simulink library "relay_housing_lib"  (Simulink 8.1)
settings: Solver=ode45  StartTime=0.0  StopTime=10.0  RelTol=1e-3
values from neighbouring files (symbols this model uses):
  Ts = 100E-6    (= 0.0001)    [BANSHEE_init.m]
undefined symbols (not defined in the file or in its folder): F1, F2, F3, generic_ethernet_cb
libraries: relay_modbus_lib x42, rtio_generic_modbus x42, rtlab x5, udp_powerfactor_lib x3, PQFV_lib x3, opal_lib x1, DMS_slave_lib x1, LoadProfiles_lib x1
(part 1 of 2)
settings Model: Creator=re25624  LastModifiedBy=g73labuser

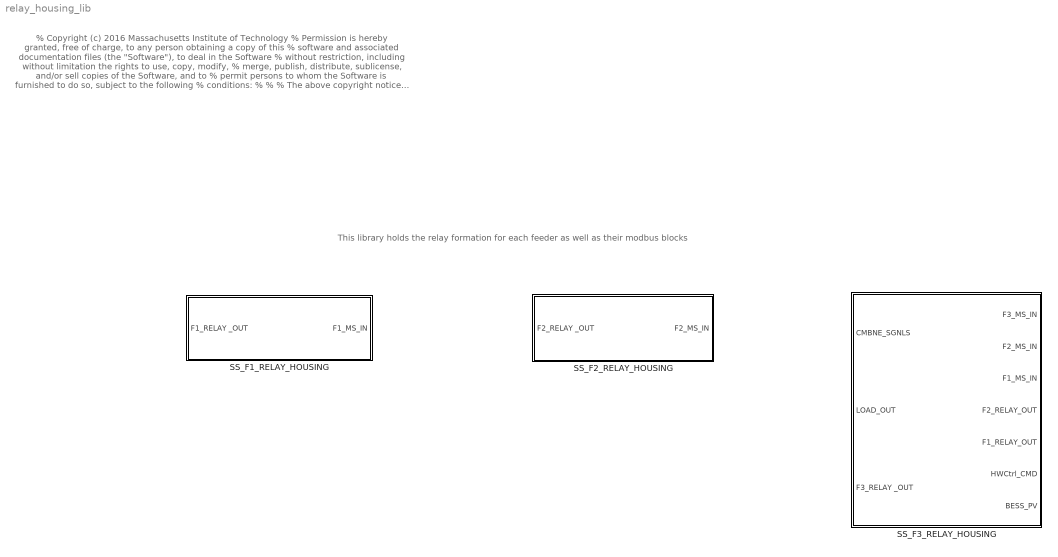
== system relay_housing_lib ==
  note: This library holds the relay formation for each feeder as well as their modbus blocks
  note: % Copyright (c) 2016 Massachusetts Institute of Technology
      | % Permission is hereby granted, free of charge, to any person obtaining a copy of this
      | % software and associated documentation files (the "Software"), to deal in the Software
      | % without restriction, including without limitation the rights to use, copy, modify,
      | % merge, publish, distribute, sublicense, and/or sell copies of the Software, and to
      | % permit persons to whom the Software is furnished to do so, subject to the following
      | % conditions:
      | %
      | %
      | % The above copyright notice and this permission notice shall be included in
      | % all copies or substantial portions of the Software.
      | %
      | % THE SOFTWARE IS PROVIDED "AS IS", WITHOUT WARRANTY OF ANY KIND, EXPRESS OR IMPLIED,
      | % INCLUDING BUT NOT LIMITED TO THE WARRANTIES OF MERCHANTABILITY, FITNESS FOR A
      | % PARTICULAR PURPOSE AND NONINFRINGEMENT. IN NO EVENT SHALL THE AUTHORS OR COPYRIGHT
      | % HOLDERS BE LIABLE FOR ANY CLAIM, DAMAGES OR OTHER LIABILITY, WHETHER IN AN ACTION
      | % OF CONTRACT, TORT OR OTHERWISE, ARISING FROM, OUT OF OR IN CONNECTION WITH THE
      | % SOFTWARE OR THE USE OR OTHER DEALINGS IN THE SOFTWARE.
      | %
      | %
      | %%
  SS_F1_RELAY_HOUSING : Subsystem
  SS_F2_RELAY_HOUSING : Subsystem
  SS_F3_RELAY_HOUSING : Subsystem

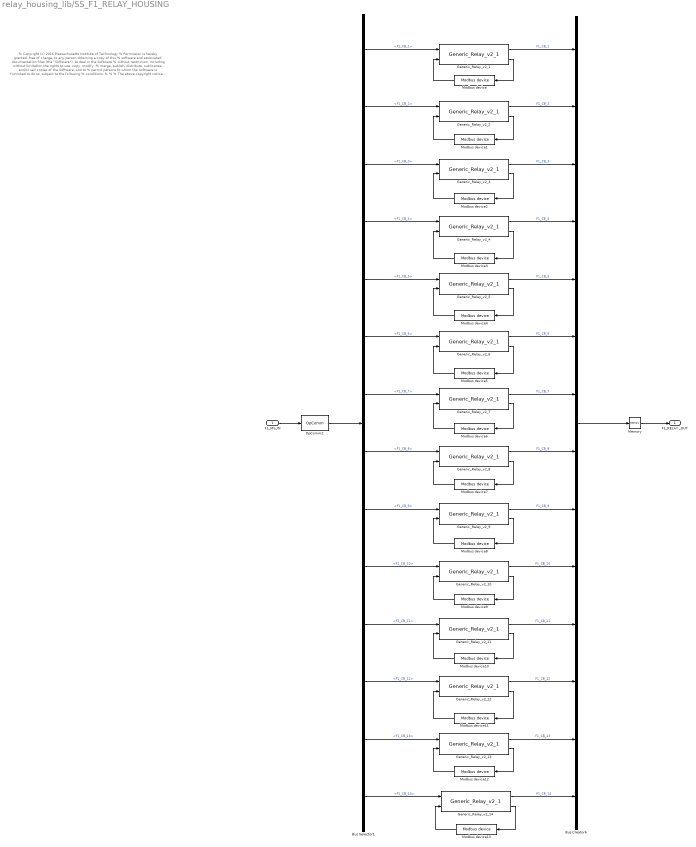
== system relay_housing_lib/SS_F1_RELAY_HOUSING ==
  note: % Copyright (c) 2016 Massachusetts Institute of Technology
      | % Permission is hereby granted, free of charge, to any person obtaining a copy of this
      | % software and associated documentation files (the "Software"), to deal in the Software
      | % without restriction, including without limitation the rights to use, copy, modify,
      | % merge, publish, distribute, sublicense, and/or sell copies of the Software, and to
      | % permit persons to whom the Software is furnished to do so, subject to the following
      | % conditions:
      | %
      | %
      | % The above copyright notice and this permission notice shall be included in
      | % all copies or substantial portions of the Software.
      | %
      | % THE SOFTWARE IS PROVIDED "AS IS", WITHOUT WARRANTY OF ANY KIND, EXPRESS OR IMPLIED,
      | % INCLUDING BUT NOT LIMITED TO THE WARRANTIES OF MERCHANTABILITY, FITNESS FOR A
      | % PARTICULAR PURPOSE AND NONINFRINGEMENT. IN NO EVENT SHALL THE AUTHORS OR COPYRIGHT
      | % HOLDERS BE LIABLE FOR ANY CLAIM, DAMAGES OR OTHER LIABILITY, WHETHER IN AN ACTION
      | % OF CONTRACT, TORT OR OTHERWISE, ARISING FROM, OUT OF OR IN CONNECTION WITH THE
      | % SOFTWARE OR THE USE OR OTHER DEALINGS IN THE SOFTWARE.
      | %
      | %
      | %%
  F1_MS_IN : Inport
  Bus Creator6 : BusCreator  Inputs=14
  Bus Selector1 : BusSelector  OutputSignals=CB_DATA.F1_CB_1,CB_DATA.F1_CB_2,CB_DATA.F1_CB_3,CB_DATA.F1_CB_4,CB_DATA.F1_CB_5,CB_DATA.F1_CB_6,CB_DATA.F1_CB_7,CB_DATA.F1_CB_8,CB_DATA.F1_CB_9,CB_DATA.F1_CB_10,CB_DATA.F1_CB_11,CB_DATA.F1_CB_12,CB_DATA.F1_CB_13,CB_DATA.F1_CB_14
  Generic_Relay_v2_1 : relay_modbus_lib/Generic_Relay_v2_1  Ts=Ts  relay_settings=[F1(1,:)]
  Generic_Relay_v2_10 : relay_modbus_lib/Generic_Relay_v2_1  Ts=Ts  relay_settings=[F1(10,:)]
  Generic_Relay_v2_11 : relay_modbus_lib/Generic_Relay_v2_1  Ts=Ts  relay_settings=[F1(11,:)]
  Generic_Relay_v2_12 : relay_modbus_lib/Generic_Relay_v2_1  Ts=Ts  relay_settings=[F1(12,:)]
  Generic_Relay_v2_13 : relay_modbus_lib/Generic_Relay_v2_1  Ts=Ts  relay_settings=[F1(13,:)]
  Generic_Relay_v2_14 : relay_modbus_lib/Generic_Relay_v2_1  Ts=Ts  relay_settings=[F1(14,:)]
  Generic_Relay_v2_2 : relay_modbus_lib/Generic_Relay_v2_1  Ts=Ts  relay_settings=[F1(2,:)]
  Generic_Relay_v2_3 : relay_modbus_lib/Generic_Relay_v2_1  Ts=Ts  relay_settings=[F1(3,:)]
  Generic_Relay_v2_4 : relay_modbus_lib/Generic_Relay_v2_1  Ts=Ts  relay_settings=[F1(4,:)]
  Generic_Relay_v2_5 : relay_modbus_lib/Generic_Relay_v2_1  Ts=Ts  relay_settings=[F1(5,:)]
  Generic_Relay_v2_6 : relay_modbus_lib/Generic_Relay_v2_1  Ts=Ts  relay_settings=[F1(6,:)]
  Generic_Relay_v2_7 : relay_modbus_lib/Generic_Relay_v2_1  Ts=Ts  relay_settings=[F1(7,:)]
  Generic_Relay_v2_8 : relay_modbus_lib/Generic_Relay_v2_1  Ts=Ts  relay_settings=[F1(8,:)]
  Generic_Relay_v2_9 : relay_modbus_lib/Generic_Relay_v2_1  Ts=Ts  relay_settings=[F1(9,:)]
  Memory : Memory
  Modbus device : rtio_generic_modbus/Modbus device  conf_name=F1_relay_cfg1.opal  conf_name_mask=F1_relay_cfg1.xls  sample_time=Ts
  Modbus device1 : rtio_generic_modbus/Modbus device  conf_name=F1_relay_cfg2.opal  conf_name_mask=F1_relay_cfg2.xls  sample_time=Ts
  Modbus device10 : rtio_generic_modbus/Modbus device  conf_name=F1_relay_cfg11.opal  conf_name_mask=F1_relay_cfg11.xls  sample_time=Ts
  Modbus device11 : rtio_generic_modbus/Modbus device  conf_name=F1_relay_cfg12.opal  conf_name_mask=F1_relay_cfg12.xls  sample_time=Ts
  Modbus device12 : rtio_generic_modbus/Modbus device  conf_name=F1_relay_cfg13.opal  conf_name_mask=F1_relay_cfg13.xls  sample_time=Ts
  Modbus device13 : rtio_generic_modbus/Modbus device  conf_name=F1_relay_cfg14.opal  conf_name_mask=F1_relay_cfg14.xls  sample_time=Ts
  Modbus device2 : rtio_generic_modbus/Modbus device  conf_name=F1_relay_cfg3.opal  conf_name_mask=F1_relay_cfg3.xls  sample_time=Ts
  Modbus device3 : rtio_generic_modbus/Modbus device  conf_name=F1_relay_cfg4.opal  conf_name_mask=F1_relay_cfg4.xls  sample_time=Ts
  Modbus device4 : rtio_generic_modbus/Modbus device  conf_name=F1_relay_cfg5.opal  conf_name_mask=F1_relay_cfg5.xls  sample_time=Ts
  Modbus device5 : rtio_generic_modbus/Modbus device  conf_name=F1_relay_cfg6.opal  conf_name_mask=F1_relay_cfg6.xls  sample_time=Ts
  Modbus device6 : rtio_generic_modbus/Modbus device  conf_name=F1_relay_cfg7.opal  conf_name_mask=F1_relay_cfg7.xls  sample_time=Ts
  Modbus device7 : rtio_generic_modbus/Modbus device  conf_name=F1_relay_cfg8.opal  conf_name_mask=F1_relay_cfg8.xls  sample_time=Ts
  Modbus device8 : rtio_generic_modbus/Modbus device  conf_name=F1_relay_cfg9.opal  conf_name_mask=F1_relay_cfg9.xls  sample_time=Ts
  Modbus device9 : rtio_generic_modbus/Modbus device  conf_name=F1_relay_cfg10.opal  conf_name_mask=F1_relay_cfg10.xls  sample_time=Ts
  OpComm2 : rtlab/OpComm  nbport=1  groupe_acq=1  subsys_rate=0  st=0  Synchronization=on  Interpolation=on  Threshold=1.0  Missed_Data=off  Sim_Time=off  Samples=off  dynSigOut=off  from_console=0  warning_done=off  writeOpCommFile=off  Offset=off
  F1_RELAY _OUT : Outport
  wires:
  Memory/1 -> F1_RELAY _OUT/1
  Bus Selector1/14 -> Generic_Relay_v2_14/1  "<F1_CB_14>"
  Generic_Relay_v2_14/1 -> Bus Creator6/14  "F1_CB_14"
  Generic_Relay_v2_14/2 -> Modbus device13/1
  Modbus device13/1 -> Generic_Relay_v2_14/2
  Generic_Relay_v2_3/1 -> Bus Creator6/3  "F1_CB_3"
  Generic_Relay_v2_4/1 -> Bus Creator6/4  "F1_CB_4"
  Generic_Relay_v2_5/1 -> Bus Creator6/5  "F1_CB_5"
  Generic_Relay_v2_6/1 -> Bus Creator6/6  "F1_CB_6"
  Generic_Relay_v2_7/1 -> Bus Creator6/7  "F1_CB_7"
  Generic_Relay_v2_8/1 -> Bus Creator6/8  "F1_CB_8"
  Generic_Relay_v2_9/1 -> Bus Creator6/9  "F1_CB_9"
  Generic_Relay_v2_10/1 -> Bus Creator6/10  "F1_CB_10"
  Generic_Relay_v2_11/1 -> Bus Creator6/11  "F1_CB_11"
  Generic_Relay_v2_12/1 -> Bus Creator6/12  "F1_CB_12"
  Generic_Relay_v2_13/1 -> Bus Creator6/13  "F1_CB_13"
  Bus Selector1/13 -> Generic_Relay_v2_13/1  "<F1_CB_13>"
  Bus Selector1/12 -> Generic_Relay_v2_12/1  "<F1_CB_12>"
  Bus Selector1/11 -> Generic_Relay_v2_11/1  "<F1_CB_11>"
  Bus Selector1/10 -> Generic_Relay_v2_10/1  "<F1_CB_10>"
  Bus Selector1/9 -> Generic_Relay_v2_9/1  "<F1_CB_9>"
  Bus Selector1/8 -> Generic_Relay_v2_8/1  "<F1_CB_8>"
  Bus Selector1/7 -> Generic_Relay_v2_7/1  "<F1_CB_7>"
  Bus Selector1/6 -> Generic_Relay_v2_6/1  "<F1_CB_6>"
  Bus Selector1/5 -> Generic_Relay_v2_5/1  "<F1_CB_5>"
  Bus Selector1/4 -> Generic_Relay_v2_4/1  "<F1_CB_4>"
  Bus Selector1/3 -> Generic_Relay_v2_3/1  "<F1_CB_3>"
  Generic_Relay_v2_2/1 -> Bus Creator6/2  "F1_CB_2"
  Bus Selector1/2 -> Generic_Relay_v2_2/1  "<F1_CB_2>"
  Bus Creator6/1 -> Memory/1
  Generic_Relay_v2_1/1 -> Bus Creator6/1  "F1_CB_1"
  Bus Selector1/1 -> Generic_Relay_v2_1/1  "<F1_CB_1>"
  F1_MS_IN/1 -> OpComm2/1
  Modbus device/1 -> Generic_Relay_v2_1/2
  Generic_Relay_v2_1/2 -> Modbus device/1
  Modbus device1/1 -> Generic_Relay_v2_2/2
  Generic_Relay_v2_2/2 -> Modbus device1/1
  Generic_Relay_v2_3/2 -> Modbus device2/1
  Modbus device2/1 -> Generic_Relay_v2_3/2
  Generic_Relay_v2_4/2 -> Modbus device3/1
  Modbus device3/1 -> Generic_Relay_v2_4/2
  Generic_Relay_v2_5/2 -> Modbus device4/1
  Modbus device4/1 -> Generic_Relay_v2_5/2
  Generic_Relay_v2_6/2 -> Modbus device5/1
  Modbus device5/1 -> Generic_Relay_v2_6/2
  Generic_Relay_v2_7/2 -> Modbus device6/1
  Modbus device6/1 -> Generic_Relay_v2_7/2
  Generic_Relay_v2_8/2 -> Modbus device7/1
  Modbus device7/1 -> Generic_Relay_v2_8/2
  Generic_Relay_v2_9/2 -> Modbus device8/1
  Modbus device8/1 -> Generic_Relay_v2_9/2
  Generic_Relay_v2_10/2 -> Modbus device9/1
  Modbus device9/1 -> Generic_Relay_v2_10/2
  Generic_Relay_v2_11/2 -> Modbus device10/1
  Modbus device10/1 -> Generic_Relay_v2_11/2
  Generic_Relay_v2_12/2 -> Modbus device11/1
  Modbus device11/1 -> Generic_Relay_v2_12/2
  Generic_Relay_v2_13/2 -> Modbus device12/1
  Modbus device12/1 -> Generic_Relay_v2_13/2
  OpComm2/1 -> Bus Selector1/1

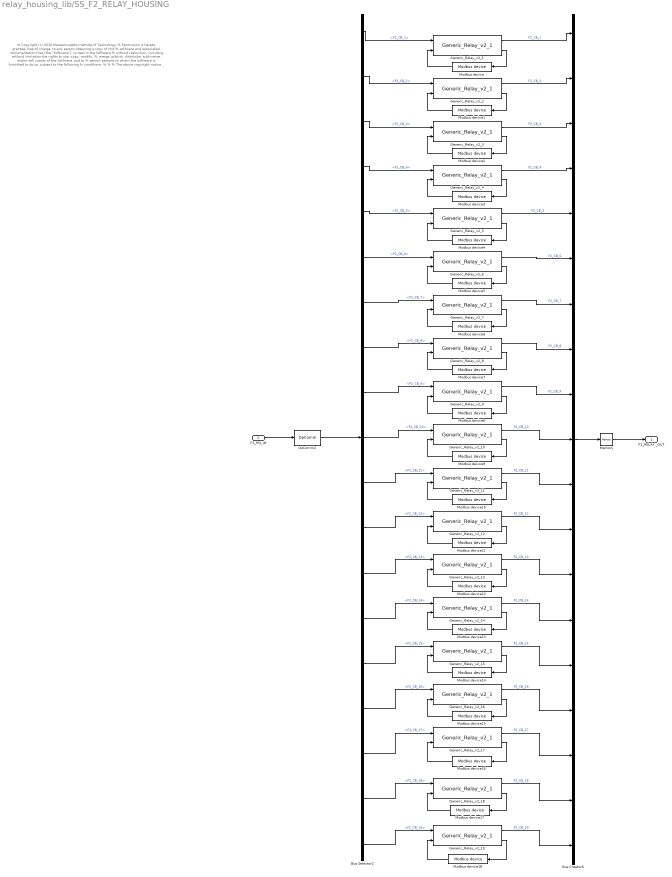
== system relay_housing_lib/SS_F2_RELAY_HOUSING ==
  note: % Copyright (c) 2016 Massachusetts Institute of Technology
      | % Permission is hereby granted, free of charge, to any person obtaining a copy of this
      | % software and associated documentation files (the "Software"), to deal in the Software
      | % without restriction, including without limitation the rights to use, copy, modify,
      | % merge, publish, distribute, sublicense, and/or sell copies of the Software, and to
      | % permit persons to whom the Software is furnished to do so, subject to the following
      | % conditions:
      | %
      | %
      | % The above copyright notice and this permission notice shall be included in
      | % all copies or substantial portions of the Software.
      | %
      | % THE SOFTWARE IS PROVIDED "AS IS", WITHOUT WARRANTY OF ANY KIND, EXPRESS OR IMPLIED,
      | % INCLUDING BUT NOT LIMITED TO THE WARRANTIES OF MERCHANTABILITY, FITNESS FOR A
      | % PARTICULAR PURPOSE AND NONINFRINGEMENT. IN NO EVENT SHALL THE AUTHORS OR COPYRIGHT
      | % HOLDERS BE LIABLE FOR ANY CLAIM, DAMAGES OR OTHER LIABILITY, WHETHER IN AN ACTION
      | % OF CONTRACT, TORT OR OTHERWISE, ARISING FROM, OUT OF OR IN CONNECTION WITH THE
      | % SOFTWARE OR THE USE OR OTHER DEALINGS IN THE SOFTWARE.
      | %
      | %
      | %%
  F2_MS_IN : Inport
  Bus Creator6 : BusCreator  Inputs=19
  Bus Selector2 : BusSelector  OutputSignals=CB_DATA.F2_CB_1,CB_DATA.F2_CB_2,CB_DATA.F2_CB_3,CB_DATA.F2_CB_4,CB_DATA.F2_CB_5,CB_DATA.F2_CB_6,CB_DATA.F2_CB_7,CB_DATA.F2_CB_8,CB_DATA.F2_CB_9,CB_DATA.F2_CB_10,CB_DATA.F2_CB_11,CB_DATA.F2_CB_12,CB_DATA.F2_CB_13,CB_DATA.F2_CB_14,CB_DATA.F2_CB_15,CB_DATA.F2_CB_16,CB_DATA.F2_CB_17,CB_DATA.F2_CB_18,CB_DATA.F2_CB_19
  Generic_Relay_v2_1 : relay_modbus_lib/Generic_Relay_v2_1  Ts=Ts  relay_settings=[F2(1,:)]
  Generic_Relay_v2_10 : relay_modbus_lib/Generic_Relay_v2_1  Ts=Ts  relay_settings=[F2(10,:)]
  Generic_Relay_v2_11 : relay_modbus_lib/Generic_Relay_v2_1  Ts=Ts  relay_settings=[F2(11,:)]
  Generic_Relay_v2_12 : relay_modbus_lib/Generic_Relay_v2_1  Ts=Ts  relay_settings=[F2(12,:)]
  Generic_Relay_v2_13 : relay_modbus_lib/Generic_Relay_v2_1  Ts=Ts  relay_settings=[F2(13,:)]
  Generic_Relay_v2_14 : relay_modbus_lib/Generic_Relay_v2_1  Ts=Ts  relay_settings=[F2(14,:)]
  Generic_Relay_v2_15 : relay_modbus_lib/Generic_Relay_v2_1  Ts=Ts  relay_settings=[F2(15,:)]
  Generic_Relay_v2_16 : relay_modbus_lib/Generic_Relay_v2_1  Ts=Ts  relay_settings=[F2(16,:)]
  Generic_Relay_v2_17 : relay_modbus_lib/Generic_Relay_v2_1  Ts=Ts  relay_settings=[F2(17,:)]
  Generic_Relay_v2_18 : relay_modbus_lib/Generic_Relay_v2_1  Ts=Ts  relay_settings=[F2(18,:)]
  Generic_Relay_v2_19 : relay_modbus_lib/Generic_Relay_v2_1  Ts=Ts  relay_settings=[F2(19,:)]
  Generic_Relay_v2_2 : relay_modbus_lib/Generic_Relay_v2_1  Ts=Ts  relay_settings=[F2(2,:)]
  Generic_Relay_v2_3 : relay_modbus_lib/Generic_Relay_v2_1  Ts=Ts  relay_settings=[F2(3,:)]
  Generic_Relay_v2_4 : relay_modbus_lib/Generic_Relay_v2_1  Ts=Ts  relay_settings=[F2(4,:)]
  Generic_Relay_v2_5 : relay_modbus_lib/Generic_Relay_v2_1  Ts=Ts  relay_settings=[F2(5,:)]
  Generic_Relay_v2_6 : relay_modbus_lib/Generic_Relay_v2_1  Ts=Ts  relay_settings=[F2(6,:)]
  Generic_Relay_v2_7 : relay_modbus_lib/Generic_Relay_v2_1  Ts=Ts  relay_settings=[F2(7,:)]
  Generic_Relay_v2_8 : relay_modbus_lib/Generic_Relay_v2_1  Ts=Ts  relay_settings=[F2(8,:)]
  Generic_Relay_v2_9 : relay_modbus_lib/Generic_Relay_v2_1  Ts=Ts  relay_settings=[F2(9,:)]
  Memory : Memory
  Modbus device : rtio_generic_modbus/Modbus device  conf_name=F2_relay_cfg1.opal  conf_name_mask=F2_relay_cfg1.xls  sample_time=Ts
  Modbus device1 : rtio_generic_modbus/Modbus device  conf_name=F2_relay_cfg2.opal  conf_name_mask=F2_relay_cfg2.xls  sample_time=Ts
  Modbus device10 : rtio_generic_modbus/Modbus device  conf_name=F2_relay_cfg11.opal  conf_name_mask=F2_relay_cfg11.xls  sample_time=Ts
  Modbus device11 : rtio_generic_modbus/Modbus device  conf_name=F2_relay_cfg12.opal  conf_name_mask=F2_relay_cfg12.xls  sample_time=Ts
  Modbus device12 : rtio_generic_modbus/Modbus device  conf_name=F2_relay_cfg13.opal  conf_name_mask=F2_relay_cfg13.xls  sample_time=Ts
  Modbus device13 : rtio_generic_modbus/Modbus device  conf_name=F2_relay_cfg14.opal  conf_name_mask=F2_relay_cfg14.xls  sample_time=Ts
  Modbus device14 : rtio_generic_modbus/Modbus device  conf_name=F2_relay_cfg15.opal  conf_name_mask=F2_relay_cfg15.xls  sample_time=Ts
  Modbus device15 : rtio_generic_modbus/Modbus device  conf_name=F2_relay_cfg16.opal  conf_name_mask=F2_relay_cfg16.xls  sample_time=Ts
  Modbus device16 : rtio_generic_modbus/Modbus device  conf_name=F2_relay_cfg17.opal  conf_name_mask=F2_relay_cfg17.xls  sample_time=Ts
  Modbus device17 : rtio_generic_modbus/Modbus device  conf_name=F2_relay_cfg18.opal  conf_name_mask=F2_relay_cfg18.xls  sample_time=Ts
  Modbus device18 : rtio_generic_modbus/Modbus device  conf_name=F2_relay_cfg19.opal  conf_name_mask=F2_relay_cfg19.xls  sample_time=Ts
  Modbus device2 : rtio_generic_modbus/Modbus device  conf_name=F2_relay_cfg3.opal  conf_name_mask=F2_relay_cfg3.xls  sample_time=Ts
  Modbus device3 : rtio_generic_modbus/Modbus device  conf_name=F2_relay_cfg4.opal  conf_name_mask=F2_relay_cfg4.xls  sample_time=Ts
  Modbus device4 : rtio_generic_modbus/Modbus device  conf_name=F2_relay_cfg5.opal  conf_name_mask=F2_relay_cfg5.xls  sample_time=Ts
  Modbus device5 : rtio_generic_modbus/Modbus device  conf_name=F2_relay_cfg6.opal  conf_name_mask=F2_relay_cfg6.xls  sample_time=Ts
  Modbus device6 : rtio_generic_modbus/Modbus device  conf_name=F2_relay_cfg7.opal  conf_name_mask=F2_relay_cfg7.xls  sample_time=Ts
  Modbus device7 : rtio_generic_modbus/Modbus device  conf_name=F2_relay_cfg8.opal  conf_name_mask=F2_relay_cfg8.xls  sample_time=Ts
  Modbus device8 : rtio_generic_modbus/Modbus device  conf_name=F2_relay_cfg9.opal  conf_name_mask=F2_relay_cfg9.xls  sample_time=Ts
  Modbus device9 : rtio_generic_modbus/Modbus device  conf_name=F2_relay_cfg10.opal  conf_name_mask=F2_relay_cfg10.xls  sample_time=Ts
  OpComm2 : rtlab/OpComm  nbport=1  groupe_acq=1  subsys_rate=0  st=0  Synchronization=on  Interpolation=on  Threshold=1.0  Missed_Data=off  Sim_Time=off  Samples=off  dynSigOut=off  from_console=0  warning_done=off  writeOpCommFile=off  Offset=off
  F2_RELAY _OUT : Outport
  wires:
  Memory/1 -> F2_RELAY _OUT/1
  Bus Selector2/18 -> Generic_Relay_v2_18/1  "<F2_CB_18>"
  Bus Selector2/19 -> Generic_Relay_v2_19/1  "<F2_CB_19>"
  Generic_Relay_v2_19/1 -> Bus Creator6/19  "F2_CB_19"
  Generic_Relay_v2_18/1 -> Bus Creator6/18  "F2_CB_18"
  Generic_Relay_v2_18/2 -> Modbus device17/1
  Modbus device17/1 -> Generic_Relay_v2_18/2
  Generic_Relay_v2_19/2 -> Modbus device18/1
  Modbus device18/1 -> Generic_Relay_v2_19/2
  Bus Selector2/17 -> Generic_Relay_v2_17/1  "<F2_CB_17>"
  Generic_Relay_v2_17/1 -> Bus Creator6/17  "F2_CB_17"
  Generic_Relay_v2_6/1 -> Bus Creator6/6  "F2_CB_6"
  Generic_Relay_v2_5/1 -> Bus Creator6/5  "F2_CB_5"
  Generic_Relay_v2_4/1 -> Bus Creator6/4  "F2_CB_4"
  Generic_Relay_v2_3/1 -> Bus Creator6/3  "F2_CB_3"
  Generic_Relay_v2_2/1 -> Bus Creator6/2  "F2_CB_2"
  Generic_Relay_v2_7/1 -> Bus Creator6/7  "F2_CB_7"
  Generic_Relay_v2_8/1 -> Bus Creator6/8  "F2_CB_8"
  Generic_Relay_v2_9/1 -> Bus Creator6/9  "F2_CB_9"
  Generic_Relay_v2_10/1 -> Bus Creator6/10  "F2_CB_10"
  Generic_Relay_v2_11/1 -> Bus Creator6/11  "F2_CB_11"
  Generic_Relay_v2_16/1 -> Bus Creator6/16  "F2_CB_16"
  Generic_Relay_v2_15/1 -> Bus Creator6/15  "F2_CB_15"
  Generic_Relay_v2_14/1 -> Bus Creator6/14  "F2_CB_14"
  Generic_Relay_v2_13/1 -> Bus Creator6/13  "F2_CB_13"
  Generic_Relay_v2_12/1 -> Bus Creator6/12  "F2_CB_12"
  Bus Selector2/16 -> Generic_Relay_v2_16/1  "<F2_CB_16>"
  Bus Selector2/15 -> Generic_Relay_v2_15/1  "<F2_CB_15>"
  Bus Selector2/14 -> Generic_Relay_v2_14/1  "<F2_CB_14>"
  Bus Selector2/13 -> Generic_Relay_v2_13/1  "<F2_CB_13>"
  Bus Selector2/12 -> Generic_Relay_v2_12/1  "<F2_CB_12>"
  Bus Selector2/11 -> Generic_Relay_v2_11/1  "<F2_CB_11>"
  Bus Selector2/10 -> Generic_Relay_v2_10/1  "<F2_CB_10>"
  Bus Selector2/9 -> Generic_Relay_v2_9/1  "<F2_CB_9>"
  Bus Selector2/8 -> Generic_Relay_v2_8/1  "<F2_CB_8>"
  Bus Selector2/7 -> Generic_Relay_v2_7/1  "<F2_CB_7>"
  Bus Selector2/6 -> Generic_Relay_v2_6/1  "<F2_CB_6>"
  Bus Selector2/5 -> Generic_Relay_v2_5/1  "<F2_CB_5>"
  Bus Selector2/4 -> Generic_Relay_v2_4/1  "<F2_CB_4>"
  Bus Selector2/3 -> Generic_Relay_v2_3/1  "<F2_CB_3>"
  Bus Selector2/2 -> Generic_Relay_v2_2/1  "<F2_CB_2>"
  Generic_Relay_v2_1/1 -> Bus Creator6/1  "F2_CB_1"
  Bus Selector2/1 -> Generic_Relay_v2_1/1  "<F2_CB_1>"
  F2_MS_IN/1 -> OpComm2/1
  Bus Creator6/1 -> Memory/1
  Generic_Relay_v2_1/2 -> Modbus device/1
  Modbus device/1 -> Generic_Relay_v2_1/2
  Generic_Relay_v2_2/2 -> Modbus device1/1
  Modbus device1/1 -> Generic_Relay_v2_2/2
  Generic_Relay_v2_3/2 -> Modbus device2/1
  Modbus device2/1 -> Generic_Relay_v2_3/2
  Generic_Relay_v2_4/2 -> Modbus device3/1
  Modbus device3/1 -> Generic_Relay_v2_4/2
  Generic_Relay_v2_5/2 -> Modbus device4/1
  Modbus device4/1 -> Generic_Relay_v2_5/2
  Modbus device5/1 -> Generic_Relay_v2_6/2
  Generic_Relay_v2_6/2 -> Modbus device5/1
  Generic_Relay_v2_7/2 -> Modbus device6/1
  Modbus device6/1 -> Generic_Relay_v2_7/2
  Generic_Relay_v2_8/2 -> Modbus device7/1
  Modbus device7/1 -> Generic_Relay_v2_8/2
  Generic_Relay_v2_9/2 -> Modbus device8/1
  Modbus device8/1 -> Generic_Relay_v2_9/2
  Generic_Relay_v2_10/2 -> Modbus device9/1
  Modbus device9/1 -> Generic_Relay_v2_10/2
  Generic_Relay_v2_11/2 -> Modbus device10/1
  Modbus device10/1 -> Generic_Relay_v2_11/2
  Generic_Relay_v2_12/2 -> Modbus device11/1
  Modbus device11/1 -> Generic_Relay_v2_12/2
  Modbus device12/1 -> Generic_Relay_v2_13/2
  Generic_Relay_v2_13/2 -> Modbus device12/1
  Generic_Relay_v2_14/2 -> Modbus device13/1
  Modbus device13/1 -> Generic_Relay_v2_14/2
  Generic_Relay_v2_15/2 -> Modbus device14/1
  Modbus device14/1 -> Generic_Relay_v2_15/2
  Generic_Relay_v2_16/2 -> Modbus device15/1
  Modbus device15/1 -> Generic_Relay_v2_16/2
  Generic_Relay_v2_17/2 -> Modbus device16/1
  Modbus device16/1 -> Generic_Relay_v2_17/2
  OpComm2/1 -> Bus Selector2/1

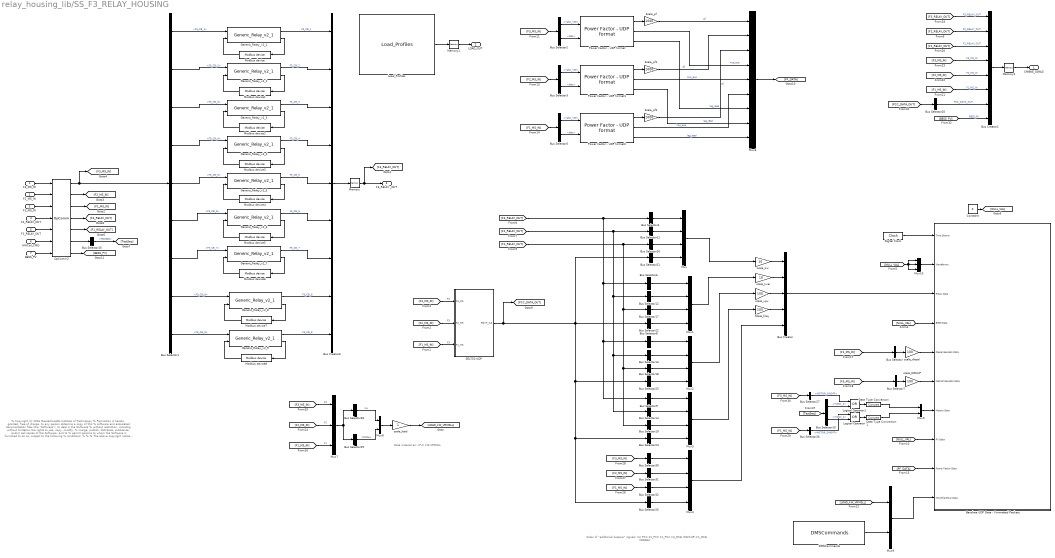
== system relay_housing_lib/SS_F3_RELAY_HOUSING ==
  note: Order of "additional breaker" signals:
      | F3_PCC
      | F2_PCC
      | F1_PCC
      | F3_GCB (NG/CHP)
      | F1_GCB (DIESEL)
  note: % Copyright (c) 2016 Massachusetts Institute of Technology
      | % Permission is hereby granted, free of charge, to any person obtaining a copy of this
      | % software and associated documentation files (the "Software"), to deal in the Software
      | % without restriction, including without limitation the rights to use, copy, modify,
      | % merge, publish, distribute, sublicense, and/or sell copies of the Software, and to
      | % permit persons to whom the Software is furnished to do so, subject to the following
      | % conditions:
      | %
      | %
      | % The above copyright notice and this permission notice shall be included in
      | % all copies or substantial portions of the Software.
      | %
      | % THE SOFTWARE IS PROVIDED "AS IS", WITHOUT WARRANTY OF ANY KIND, EXPRESS OR IMPLIED,
      | % INCLUDING BUT NOT LIMITED TO THE WARRANTIES OF MERCHANTABILITY, FITNESS FOR A
      | % PARTICULAR PURPOSE AND NONINFRINGEMENT. IN NO EVENT SHALL THE AUTHORS OR COPYRIGHT
      | % HOLDERS BE LIABLE FOR ANY CLAIM, DAMAGES OR OTHER LIABILITY, WHETHER IN AN ACTION
      | % OF CONTRACT, TORT OR OTHERWISE, ARISING FROM, OUT OF OR IN CONNECTION WITH THE
      | % SOFTWARE OR THE USE OR OTHER DEALINGS IN THE SOFTWARE.
      | %
      | %
      | %%
  note: Data ordered as:
      | I-P-C
      | kW-VRMSLL
  F3_MS_IN : Inport
  F2_MS_IN : Inport  Port=2
  F1_MS_IN : Inport  Port=3
  F2_RELAY_OUT : Inport  Port=4
  F1_RELAY_OUT : Inport  Port=5
  HWCtrl_CMD : Inport  Port=6
  BESS_PV : Inport  Port=7
  Banshee UDP Data - Formatted Packets : Subsystem  mask(UDP Data Block){ProfileID=2, NumOfWaveforms=[3, 1, 1], NumOfRelays=[47, [10, 10, 100, 100]], NumOfBatteries=0, NumOfDieselGensets=[1, [100, 100]], NumOfNGCHPGensets=[1, [100, 100, 100, 100, 100, 100, 100, 100, 100]], NumOfMotors=2, NumOfPVs=0, NumOfPF=[3, 1000], NumOfMiscellaneousDataScales=2, NumOfMiscellaneousDataSignalsScales=[[36, 1], [8, 1]]}
      mask prompts: ProfileID "Profile ID"; NumOfWaveforms "Waveform Data"; NumOfRelays "Relay Data"; NumOfBatteries "# of Batteries"; NumOfDieselGensets "Diesel Gensets Data"; NumOfNGCHPGensets "NG-CHP Gensets Data"; NumOfMotors "# of Motors"; NumOfPVs "# of PVs"; NumOfPF "Power Factor Data"; NumOfMiscellaneousDataScales "Misc. Data - No. of Scale Factors"; NumOfMiscellaneousDataSignalsScales "Misc. - No. Signals and Scale Values"
      mask help:
      | * All signal scaling/modifications should be external to this block
      |
      | Profile ID: (1-Sheriff, 2-Banshee, 3-Canary, 4-Siren)
      |
      | Waveforms Data: No. of per phase waveforms sent at 5Hz rate, point per waveforms [dt=80us, 208; dt=100us, 166], and scaling factor.
      | -Input format: [No. of waveforms, No. of data-points, scale]
      | -Ex:[3, 166, 100]
      |
      | Relay Data: No. of relays feeding packet data to breakers in display - mapped/indexed in ascending order
      | -Packet order: Active power(kW), reactive power(kVAR), voltage(per-unit), frequency (Hz), breaker status (1:closed, 0:open)
      | -Input format: [No. of Relays, [scale_kW, scale_kVAR, scale_Vpu, scale_Hz]]
      | -Ex:[4, [10, 10, 100, 100]]
      |
      | No. of Batteries: TBD
      | -Ex: [0]
      |
      | No. of Diesel Gensets: No. of diesel gensets in the system feeding data to the display.
      | -Packet order: terminal voltage(per-unit), fuel consumption (Gals/hr)
      | -Input format: [No. of gensets, [scale_Vpu, scale_fuel]]
      | -Ex: [0, [1,1]]
      |
      | No. of NG/CHP Gensets: No. of NGCHP gensets in the system feeding data to the display.
      | -Packet order: Terminal Vpu, Temp Actual, Heat Recovered, Fuel usage, CHP CO2, Heat from boiler, CHP heat contribution, Boiler Nm^3/hr, Boiler lbm/hr CO2
      | -Ex: [1, [100,100,100,100,100,100,100,100,100]]
      |
      | Motors Data: No. of motors monitored in the system. Currently, only looking at motor on/off state.
      | -Input format: [No. of motors]
      | -Ex: [1]
      |
      | No. of PV: TBD
      | -Ex: [0]
      |
      | Power Factor Data: No. of power factors to be displayed in the system and scale value. The same scale factor will be applied to all power factors.
      | -Packet order: power factor, import/export, lagging/leading
      | -Input format: [No. of Power Factors, scale_pf]
      | -Ex:[1, 1000]
      |
      | Misc. Data - No. of Scale factor: No. of scale factors to be applied to each signal-set.
      | -Ex: [3]
      |
      | Misc. Data - No. of Signals and Scale Values: Size of signal set and scale value to be applied to the signal-set.
      | -Ex: [[1, 1000], [6, 100], [3, 10]]
  Bus Creator : BusCreator  Inputs=5
  Bus Creator1 : BusCreator  Inputs=8
  Bus Creator6 : BusCreator  Inputs=9
  Bus Selector : BusSelector  OutputSignals=DIESEL_DATA.Gen2_meas.gal_per_hr,DIESEL_DATA.DIESEL_GCB.Vpu  OutputAsBus=on
  Bus Selector1 : BusSelector  OutputSignals=CB_DATA.F3_CB_1,CB_DATA.F3_CB_2,CB_DATA.F3_CB_3,CB_DATA.F3_CB_4,CB_DATA.F3_CB_5,CB_DATA.F3_CB_6,CB_DATA.F3_CB_7,CB_DATA.F3_CB_8,CB_DATA.F3_CB_9
  Bus Selector10 : BusSelector  OutputSignals=motor_2,motor_1
  Bus Selector11 : BusSelector  OutputSignals=F2_CB_1.m.kw,F2_CB_2.m.kw,F2_CB_3.m.kw,F2_CB_4.m.kw,F2_CB_5.m.kw,F2_CB_6.m.kw,F2_CB_7.m.kw,F2_CB_8.m.kw,F2_CB_9.m.kw,F2_CB_10.m.kw,F2_CB_11.m.kw,F2_CB_12.m.kw,F2_CB_13.m.kw,F2_CB_14.m.kw,F2_CB_15.m.kw,F2_CB_16.m.kw,F2_CB_17.m.kw,F2_CB_18.m.kw,F2_CB_19.m.kw  OutputAsBus=on
  Bus Selector12 : BusSelector  OutputSignals=F2_CB_1.m.kvar,F2_CB_2.m.kvar,F2_CB_3.m.kvar,F2_CB_4.m.kvar,F2_CB_5.m.kvar,F2_CB_6.m.kvar,F2_CB_7.m.kvar,F2_CB_8.m.kvar,F2_CB_9.m.kvar,F2_CB_10.m.kvar,F2_CB_11.m.kvar,F2_CB_12.m.kvar,F2_CB_13.m.kvar,F2_CB_14.m.kvar,F2_CB_15.m.kvar,F2_CB_16.m.kvar,F2_CB_17.m.kvar,F2_CB_18.m.kvar,F2_CB_19.m.kvar  OutputAsBus=on
  Bus Selector13 : BusSelector  OutputSignals=F2_CB_1.m.Vpu,F2_CB_2.m.Vpu,F2_CB_3.m.Vpu,F2_CB_4.m.Vpu,F2_CB_5.m.Vpu,F2_CB_6.m.Vpu,F2_CB_7.m.Vpu,F2_CB_8.m.Vpu,F2_CB_9.m.Vpu,F2_CB_10.m.Vpu,F2_CB_11.m.Vpu,F2_CB_12.m.Vpu,F2_CB_13.m.Vpu,F2_CB_14.m.Vpu,F2_CB_15.m.Vpu,F2_CB_16.m.Vpu,F2_CB_17.m.Vpu,F2_CB_18.m.Vpu,F2_CB_19.m.Vpu  OutputAsBus=on
  Bus Selector14 : BusSelector  OutputSignals=F2_CB_1.m.Hz,F2_CB_2.m.Hz,F2_CB_3.m.Hz,F2_CB_4.m.Hz,F2_CB_5.m.Hz,F2_CB_6.m.Hz,F2_CB_7.m.Hz,F2_CB_8.m.Hz,F2_CB_9.m.Hz,F2_CB_10.m.Hz,F2_CB_11.m.Hz,F2_CB_12.m.Hz,F2_CB_13.m.Hz,F2_CB_14.m.Hz,F2_CB_15.m.Hz,F2_CB_16.m.Hz,F2_CB_17.m.Hz,F2_CB_18.m.Hz,F2_CB_19.m.Hz  OutputAsBus=on
  Bus Selector15 : BusSelector  OutputSignals=TestSeq
  Bus Selector16 : BusSelector  OutputSignals=F1_CB_1.m.kw,F1_CB_2.m.kw,F1_CB_3.m.kw,F1_CB_4.m.kw,F1_CB_5.m.kw,F1_CB_6.m.kw,F1_CB_7.m.kw,F1_CB_8.m.kw,F1_CB_9.m.kw,F1_CB_10.m.kw,F1_CB_11.m.kw,F1_CB_12.m.kw,F1_CB_13.m.kw,F1_CB_14.m.kw  OutputAsBus=on
  Bus Selector17 : BusSelector  OutputSignals=F1_CB_1.m.kvar,F1_CB_2.m.kvar,F1_CB_3.m.kvar,F1_CB_4.m.kvar,F1_CB_5.m.kvar,F1_CB_6.m.kvar,F1_CB_7.m.kvar,F1_CB_8.m.kvar,F1_CB_9.m.kvar,F1_CB_10.m.kvar,F1_CB_12.m.kvar,F1_CB_11.m.kvar,F1_CB_13.m.kvar,F1_CB_14.m.kvar  OutputAsBus=on
  Bus Selector18 : BusSelector  OutputSignals=F1_CB_1.m.Vpu,F1_CB_2.m.Vpu,F1_CB_3.m.Vpu,F1_CB_4.m.Vpu,F1_CB_5.m.Vpu,F1_CB_6.m.Vpu,F1_CB_7.m.Vpu,F1_CB_8.m.Vpu,F1_CB_9.m.Vpu,F1_CB_10.m.Vpu,F1_CB_11.m.Vpu,F1_CB_12.m.Vpu,F1_CB_13.m.Vpu,F1_CB_14.m.Vpu  OutputAsBus=on
  Bus Selector19 : BusSelector  OutputSignals=F1_CB_1.m.Hz,F1_CB_2.m.Hz,F1_CB_3.m.Hz,F1_CB_4.m.Hz,F1_CB_5.m.Hz,F1_CB_6.m.Hz,F1_CB_7.m.Hz,F1_CB_8.m.Hz,F1_CB_9.m.Hz,F1_CB_10.m.Hz,F1_CB_11.m.Hz,F1_CB_12.m.Hz,F1_CB_13.m.Hz,F1_CB_14.m.Hz  OutputAsBus=on
  Bus Selector2 : BusSelector  OutputSignals=CB_DATA.F3_PCC.Vabc_line,CB_DATA.F3_PCC.Iabc
  Bus Selector20 : BusSelector  OutputSignals=F1_PCC,F2_PCC,F3_PCC  OutputAsBus=on
  Bus Selector21 : BusSelector  OutputSignals=F3_PCC.kw,F2_PCC.kw,F1_PCC.kw,F3_MS.NG_CHP_DATA.NG_CHP_GCB.kw,F1_MS.DIESEL_DATA.DIESEL_GCB.kw  OutputAsBus=on
  Bus Selector22 : BusSelector  OutputSignals=F3_PCC.kvar,F2_PCC.kvar,F1_PCC.kvar,F3_MS.NG_CHP_DATA.NG_CHP_GCB.kvar,F1_MS.DIESEL_DATA.DIESEL_GCB.kvar  OutputAsBus=on
  Bus Selector23 : BusSelector  OutputSignals=F3_PCC.Vpu,F2_PCC.Vpu,F1_PCC.Vpu,F3_MS.NG_CHP_DATA.NG_CHP_GCB.Vpu,F1_MS.DIESEL_DATA.DIESEL_GCB.Vpu  OutputAsBus=on
  Bus Selector24 : BusSelector  OutputSignals=F3_PCC.Freq,F2_PCC.Freq,F1_PCC.Freq,F3_MS.NG_CHP_DATA.NG_CHP_GCB.Freq,F1_MS.DIESEL_DATA.DIESEL_GCB.Freq  OutputAsBus=on
  Bus Selector25 : BusSelector  OutputSignals=F3_PCC.cb_ms.Status,F2_PCC.cb_ms.Status,F1_PCC.cb_ms.Status,F3_MS.NG_CHP_DATA.NG_CHP_GCB.cb_ms.Status,F1_MS.DIESEL_DATA.DIESEL_GCB.cb_ms.Status  OutputAsBus=on
  Bus Selector26 : BusSelector  OutputSignals=MOTOR_ONOFF
  Bus Selector27 : BusSelector  OutputSignals=MOTOR_ONOFF
  Bus Selector28 : BusSelector  OutputSignals=F1.LOAD_DATA.F1_I1.kw,F1.LOAD_DATA.F1_I2.kw,F2.LOAD_DATA.F2_I3.kw,F2.LOAD_DATA.F2_I4.kw,F2.LOAD_DATA.F2_I5.kw,F3.LOAD_DATA.F3_I6.kw,F1.LOAD_DATA.F1_P1.kw,F2.LOAD_DATA.F2_P2.kw,F2.LOAD_DATA.F2_P3.kw,F3.LOAD_DATA.F3_P4.kw,F2.LOAD_DATA.F2_P5.kw,F3.LOAD_DATA.F3_P6.kw,F1.LOAD_DATA.F1_C1.kw,F1.LOAD_DATA.F1_C2.kw,F2.LOAD_DATA.F2_C3.kw,F2.LOAD_DATA.F2_C4.kw,F3.LOAD_DATA.F3_C5.kw,F3.LOAD_DATA.F3_C6.kw  OutputAsBus=on
  Bus Selector29 : BusSelector  OutputSignals=F1.LOAD_DATA.F1_I1.VRMSLL,F1.LOAD_DATA.F1_I2.VRMSLL,F2.LOAD_DATA.F2_I3.VRMSLL,F2.LOAD_DATA.F2_I4.VRMSLL,F2.LOAD_DATA.F2_I5.VRMSLL,F3.LOAD_DATA.F3_I6.VRMSLL,F1.LOAD_DATA.F1_P1.VRMSLL,F2.LOAD_DATA.F2_P2.VRMSLL,F2.LOAD_DATA.F2_P3.VRMSLL,F3.LOAD_DATA.F3_P4.VRMSLL,F2.LOAD_DATA.F2_P5.VRMSLL,F3.LOAD_DATA.F3_P6.VRMSLL,F1.LOAD_DATA.F1_C1.VRMSLL,F1.LOAD_DATA.F1_C2.VRMSLL,F2.LOAD_DATA.F2_C3.VRMSLL,F2.LOAD_DATA.F2_C4.VRMSLL,F3.LOAD_DATA.F3_C5.VRMSLL,F3.LOAD_DATA.F3_C6.VRMSLL  OutputAsBus=on
  Bus Selector3 : BusSelector  OutputSignals=CB_DATA.F2_PCC.Vabc_line,CB_DATA.F2_PCC.Iabc
  Bus Selector30 : BusSelector  OutputSignals=CB_DATA.F3_CB_1.Status,CB_DATA.F3_CB_2.Status,CB_DATA.F3_CB_3.Status,CB_DATA.F3_CB_4.Status,CB_DATA.F3_CB_5.Status,CB_DATA.F3_CB_6.Status,CB_DATA.F3_CB_7.Status,CB_DATA.F3_CB_8.Status,CB_DATA.F3_CB_9.Status  OutputAsBus=on
  Bus Selector31 : BusSelector  OutputSignals=CB_DATA.F2_CB_1.Status,CB_DATA.F2_CB_2.Status,CB_DATA.F2_CB_3.Status,CB_DATA.F2_CB_4.Status,CB_DATA.F2_CB_5.Status,CB_DATA.F2_CB_6.Status,CB_DATA.F2_CB_7.Status,CB_DATA.F2_CB_8.Status,CB_DATA.F2_CB_9.Status,CB_DATA.F2_CB_10.Status,CB_DATA.F2_CB_11.Status,CB_DATA.F2_CB_12.Status,CB_DATA.F2_CB_13.Status,CB_DATA.F2_CB_14.Status,CB_DATA.F2_CB_15.Status,CB_DATA.F2_CB_16.Status,CB_DATA.F2_CB_17.Status,CB_DATA.F2_CB_18.Status,CB_DATA.F2_CB_19.Status  OutputAsBus=on
  Bus Selector32 : BusSelector  OutputSignals=CB_DATA.F1_CB_1.Status,CB_DATA.F1_CB_2.Status,CB_DATA.F1_CB_3.Status,CB_DATA.F1_CB_4.Status,CB_DATA.F1_CB_5.Status,CB_DATA.F1_CB_6.Status,CB_DATA.F1_CB_7.Status,CB_DATA.F1_CB_8.Status,CB_DATA.F1_CB_9.Status,CB_DATA.F1_CB_10.Status,CB_DATA.F1_CB_11.Status,CB_DATA.F1_CB_12.Status,CB_DATA.F1_CB_13.Status,CB_DATA.F1_CB_14.Status  OutputAsBus=on
  Bus Selector4 : BusSelector  OutputSignals=F3_CB_1.m.kw,F3_CB_2.m.kw,F3_CB_3.m.kw,F3_CB_4.m.kw,F3_CB_5.m.kw,F3_CB_6.m.kw,F3_CB_7.m.kw,F3_CB_8.m.kw,F3_CB_9.m.kw  OutputAsBus=on
  Bus Selector5 : BusSelector  OutputSignals=CB_DATA.F1_PCC.Vabc_line,CB_DATA.F1_PCC.Iabc
  Bus Selector6 : BusSelector  OutputSignals=F3_CB_1.m.kvar,F3_CB_2.m.kvar,F3_CB_3.m.kvar,F3_CB_4.m.kvar,F3_CB_5.m.kvar,F3_CB_6.m.kvar,F3_CB_7.m.kvar,F3_CB_8.m.kvar,F3_CB_9.m.kvar  OutputAsBus=on
  Bus Selector7 : BusSelector  OutputSignals=NG_CHP_DATA.NG_CHP_GCB.Vpu,NG_CHP_DATA.CHPData.TempActual,NG_CHP_DATA.CHPData.Thermal data.Heat Recovered; MBtu/hr,NG_CHP_DATA.CHPData.Thermal data.Nm^3 per hour NG fuel usage,NG_CHP_DATA.CHPData.Thermal data.CO2 lbm/hr,NG_CHP_DATA.CHPData.HeatFromBoiler MBtu/hr,NG_CHP_DATA.CHPData.CHPHeatContribution MBtu/hr,NG_CHP_DATA.CHPData.Boiler_Nm^3/hr ,NG_CHP_DATA.CHPData.Boiler lbm/hr CO2  OutputAsBus=on
  Bus Selector8 : BusSelector  OutputSignals=F3_CB_1.m.Vpu,F3_CB_2.m.Vpu,F3_CB_3.m.Vpu,F3_CB_4.m.Vpu,F3_CB_5.m.Vpu,F3_CB_6.m.Vpu,F3_CB_7.m.Vpu,F3_CB_8.m.Vpu,F3_CB_9.m.Vpu  OutputAsBus=on
  Bus Selector9 : BusSelector  OutputSignals=F3_CB_1.m.Hz,F3_CB_2.m.Hz,F3_CB_3.m.Hz,F3_CB_4.m.Hz,F3_CB_5.m.Hz,F3_CB_6.m.Hz,F3_CB_7.m.Hz,F3_CB_8.m.Hz,F3_CB_9.m.Hz  OutputAsBus=on
  Constant : Constant  Value=0
  DMSCommands : DMS_slave_lib/DMSCommands
  Data Type Conversion : DataTypeConversion
  Data Type Conversion1 : DataTypeConversion
  Digital Clock : DigitalClock  SampleTime=Ts
  Generic_Relay_v2_1 : relay_modbus_lib/Generic_Relay_v2_1  Ts=Ts  relay_settings=[F3(1,:)]
  Generic_Relay_v2_2 : relay_modbus_lib/Generic_Relay_v2_1  Ts=Ts  relay_settings=[F3(2,:)]
  Generic_Relay_v2_3 : relay_modbus_lib/Generic_Relay_v2_1  Ts=Ts  relay_settings=[F3(3,:)]
  Generic_Relay_v2_4 : relay_modbus_lib/Generic_Relay_v2_1  Ts=Ts  relay_settings=[F3(4,:)]
  Generic_Relay_v2_5 : relay_modbus_lib/Generic_Relay_v2_1  Ts=Ts  relay_settings=[F3(5,:)]
  Generic_Relay_v2_6 : relay_modbus_lib/Generic_Relay_v2_1  Ts=Ts  relay_settings=[F3(6,:)]
  Generic_Relay_v2_7 : relay_modbus_lib/Generic_Relay_v2_1  Ts=Ts  relay_settings=[F3(7,:)]
  Generic_Relay_v2_8 : relay_modbus_lib/Generic_Relay_v2_1  Ts=Ts  relay_settings=[F3(8,:)]
  Generic_Relay_v2_9 : relay_modbus_lib/Generic_Relay_v2_1  Ts=Ts  relay_settings=[F3(9,:)]
  Load_Profiles : LoadProfiles_lib/Load_Profiles
  Logical Operator : Logic  Operator=OR  AllPortsSameDT=off  OutDataTypeStr=boolean
  Logical Operator1 : Logic  Operator=OR  AllPortsSameDT=off  OutDataTypeStr=boolean
  Memory : Memory
  Memory1 : Memory
  Memory2 : Memory
  Modbus device : rtio_generic_modbus/Modbus device  conf_name=F3_relay_cfg1.opal  conf_name_mask=F3_relay_cfg1.xls  sample_time=Ts
  Modbus device1 : rtio_generic_modbus/Modbus device  conf_name=F3_relay_cfg2.opal  conf_name_mask=F3_relay_cfg2.xls  sample_time=Ts
  Modbus device2 : rtio_generic_modbus/Modbus device  conf_name=F3_relay_cfg3.opal  conf_name_mask=F3_relay_cfg3.xls  sample_time=Ts
  Modbus device3 : rtio_generic_modbus/Modbus device  conf_name=F3_relay_cfg4.opal  conf_name_mask=F3_relay_cfg4.xls  sample_time=Ts
  Modbus device4 : rtio_generic_modbus/Modbus device  conf_name=F3_relay_cfg5.opal  conf_name_mask=F3_relay_cfg5.xls  sample_time=Ts
  Modbus device5 : rtio_generic_modbus/Modbus device  conf_name=F3_relay_cfg6.opal  conf_name_mask=F3_relay_cfg6.xls  sample_time=Ts
  Modbus device6 : rtio_generic_modbus/Modbus device  conf_name=F3_relay_cfg7.opal  conf_name_mask=F3_relay_cfg7.xls  sample_time=Ts
  Modbus device7 : rtio_generic_modbus/Modbus device  conf_name=F3_relay_cfg8.opal  conf_name_mask=F3_relay_cfg8.xls  sample_time=Ts
  Modbus device8 : rtio_generic_modbus/Modbus device  conf_name=F3_relay_cfg9.opal  conf_name_mask=F3_relay_cfg9.xls  sample_time=Ts
  Mux{,1..4} (5 alike) : Mux
  Mux10 : Mux  Inputs=3
  Mux5 : Mux  Inputs=2
  Mux6 : Mux  Inputs=9
  Mux7 : Mux  Inputs=3
  Mux8 : Mux  Inputs=2
  Mux9 : Mux  Inputs=2
  OpComm2 : rtlab/OpComm  nbport=7  groupe_acq=1  subsys_rate=0  st=0  Synchronization=on  Interpolation=on  Threshold=1.0  Missed_Data=off  Sim_Time=off  Samples=off  dynSigOut=off  from_console=0  warning_done=off  writeOpCommFile=off  Offset=off
  Power Factor - UDP format : udp_powerfactor_lib/Power Factor - UDP format
  Power Factor - UDP format1 : udp_powerfactor_lib/Power Factor - UDP format
  Power Factor - UDP format2 : udp_powerfactor_lib/Power Factor - UDP format
  SEL751-UDP : Subsystem
  Scale_freq : Gain  Gain=100
  Scale_pf : Gain  Gain=1000
  Scale_pf1 : Gain  Gain=1000
  Scale_pf2 : Gain  Gain=1000
  scale_NGCHP : Gain  Gain=100
  scale_diesel : Gain  Gain=100
  scale_kvar : Gain  Gain=10
  scale_kw : Gain  Gain=10
  scale_load : Gain
  scale_vpu : Gain  Gain=100
  CMBNE_SGNLS : Outport
  LOAD_OUT : Outport  Port=2
  F3_RELAY _OUT : Outport  Port=3
  wires:
  [BESS_PV] -> Bus Creator1/8  "BESS_PV"
  OpComm2/7 -> [BESS_PV]
  BESS_PV/1 -> OpComm2/7
  Bus Selector20/1 -> Bus Creator1/7  "PCC_DATA_OUT"
  [PCC_DATA_OUT] -> Bus Selector20/1
  Data Type Conversion/1 -> Mux5/1
  Data Type Conversion1/1 -> Mux5/2
  Logical Operator/1 -> Data Type Conversion1/1
  Logical Operator1/1 -> Data Type Conversion/1
  [F3_MS_IN] -> Bus Selector27/1
  [F1_MS_IN] -> Bus Selector26/1
  Bus Selector10/1 -> Logical Operator1/2  "<motor_2>"
  Bus Selector10/2 -> Logical Operator/2  "<motor_1>"
  Bus Selector15/1 -> [TestSeq]  "<TestSeq>"
  OpComm2/6 -> Bus Selector15/1
  HWCtrl_CMD/1 -> OpComm2/6
  [TestSeq] -> Bus Selector10/1
  Mux9/1 -> Banshee UDP Data - Formatted Packets/10(Miscellaneous Data)
  DMSCommands/1 -> Mux9/2
  Bus Selector30/1 -> Mux4/1
  Bus Selector32/1 -> Mux4/3
  Bus Selector31/1 -> Mux4/2
  [F1_MS_IN] -> Bus Selector32/1
  [F2_MS_IN] -> Bus Selector31/1
  [F3_MS_IN] -> Bus Selector30/1
  scale_load/1 -> [LOAD_kW_VRMSLL]
  Mux8/1 -> scale_load/1
  Bus Selector29/1 -> Mux8/2  "VRMSLL"
  Bus Selector28/1 -> Mux8/1  "kw"
  Mux7/1 -> Bus Selector29/1, Bus Selector28/1
  [F1_MS_IN] -> Mux7/3  "F1"
  [F2_MS_IN] -> Mux7/2  "F2"
  [F3_MS_IN] -> Mux7/1  "F3"
  Power Factor - UDP format2/3 -> Mux6/9  "lag_lead"
  Power Factor - UDP format1/3 -> Mux6/8  "lag_lead"
  Power Factor - UDP format/3 -> Mux6/7  "lag_lead"
  Power Factor - UDP format2/2 -> Mux6/6  "imp_exp"
  Power Factor - UDP format1/2 -> Mux6/5  "imp_exp"
  Power Factor - UDP format/2 -> Mux6/4  "imp_exp"
  Scale_pf2/1 -> Mux6/3  "pf"
  Scale_pf1/1 -> Mux6/2  "pf"
  Scale_pf/1 -> Mux6/1  "pf"
  Mux6/1 -> [PF_DATA]
  Digital Clock/1 -> Banshee UDP Data - Formatted Packets/1(Time Stamp)
  Mux5/1 -> Banshee UDP Data - Formatted Packets/7(Motors Data)
  Bus Selector26/1 -> Logical Operator/1  "<MOTOR_ONOFF>"
  Bus Selector27/1 -> Logical Operator1/1  "<MOTOR_ONOFF>"
  [F2_MS_IN] -> Bus Creator1/5  "F2_MS_IN"
  [F3_MS_IN] -> Bus Creator1/4  "F3_MS_IN"
  [F3_RELAY_OUT] -> Bus Creator1/1  "F3_RELAY_OUT"
  [F1_RELAY_OUT] -> Bus Creator1/3  "F1_RELAY_OUT"
  [F2_RELAY_OUT] -> Bus Creator1/2  "F2_RELAY_OUT"
  [F1_MS_IN] -> Bus Creator1/6  "F1_MS_IN"
  Bus Creator1/1 -> Memory2/1
  Memory2/1 -> CMBNE_SGNLS/1
  Bus Selector25/1 -> Mux4/4
  Bus Selector24/1 -> Mux3/4
  Bus Selector23/1 -> Mux2/4
  Bus Selector22/1 -> Mux1/4
  SEL751-UDP/1(PQVF_out) -> Bus Selector22/1, Bus Selector23/1, Bus Selector24/1, Bus Selector25/1, Bus Selector21/1, [PCC_DATA_OUT]
  Bus Selector21/1 -> Mux/4
  scale_NGCHP/1 -> Banshee UDP Data - Formatted Packets/6(NGCHP Gensets Data)
  Bus Selector7/1 -> scale_NGCHP/1
  scale_diesel/1 -> Banshee UDP Data - Formatted Packets/5(Diesel Gensets Data)
  [F3_MS_IN] -> Bus Selector7/1
  Bus Selector/1 -> scale_diesel/1
  [F1_MS_IN] -> Bus Selector/1
  [F1_RELAY_OUT] -> Bus Selector16/1, Bus Selector19/1, Bus Selector18/1, Bus Selector17/1
  Bus Selector16/1 -> Mux/3
  Bus Selector17/1 -> Mux1/3
  Bus Selector18/1 -> Mux2/3
  Bus Selector19/1 -> Mux3/3
  [F2_RELAY_OUT] -> Bus Selector11/1, Bus Selector12/1, Bus Selector13/1, Bus Selector14/1
  Bus Selector14/1 -> Mux3/2
  Bus Selector13/1 -> Mux2/2
  Bus Selector11/1 -> Mux/2
  Bus Selector12/1 -> Mux1/2
  [F3_RELAY_OUT] -> Bus Selector4/1, Bus Selector6/1, Bus Selector8/1, Bus Selector9/1
  Bus Selector9/1 -> Mux3/1
  Bus Selector8/1 -> Mux2/1
  Bus Selector6/1 -> Mux1/1
  Bus Selector4/1 -> Mux/1
  [PF_DATA] -> Banshee UDP Data - Formatted Packets/9(Power Factor Data)
  Bus Selector5/2 -> Power Factor - UDP format2/2  "<Iabc>"
  Bus Selector5/1 -> Power Factor - UDP format2/1  "<Vabc_line>"
  [F1_MS_IN] -> Bus Selector5/1
  Power Factor - UDP format2/1 -> Scale_pf2/1
  Bus Selector3/2 -> Power Factor - UDP format1/2  "<Iabc>"
  Bus Selector3/1 -> Power Factor - UDP format1/1  "<Vabc_line>"
  [F2_MS_IN] -> Bus Selector3/1
  Power Factor - UDP format1/1 -> Scale_pf1/1
  [LOAD_kW_VRMSLL] -> Mux9/1
  Bus Selector2/2 -> Power Factor - UDP format/2  "<Iabc>"
  Bus Selector2/1 -> Power Factor - UDP format/1  "<Vabc_line>"
  [F3_MS_IN] -> Bus Selector2/1
  Power Factor - UDP format/1 -> Scale_pf/1
  [NULL_VAL] -> Banshee UDP Data - Formatted Packets/8(PV Data)
  [NULL_VAL] -> Banshee UDP Data - Formatted Packets/4(BESS Data)
  Mux4/1 -> Bus Creator/5
  Mux3/1 -> Scale_freq/1
  Mux2/1 -> scale_vpu/1
  Mux1/1 -> scale_kvar/1
  Mux/1 -> scale_kw/1
  scale_vpu/1 -> Bus Creator/3
  Scale_freq/1 -> Bus Creator/4
  scale_kvar/1 -> Bus Creator/2
  scale_kw/1 -> Bus Creator/1
  Bus Creator/1 -> Banshee UDP Data - Formatted Packets/3(Relay Data)
  Constant/1 -> [NULL_VAL]
  Mux10/1 -> Banshee UDP Data - Formatted Packets/2(Waveforms)
  [NULL_VAL] -> Mux10/2, Mux10/1, Mux10/3
  [F1_MS_IN] -> SEL751-UDP/3(F1_MS)  "F3"
  [F2_MS_IN] -> SEL751-UDP/2(F2_MS)  "F3"
  [F3_MS_IN] -> SEL751-UDP/1(F3_MS)  "F3"
  F1_MS_IN/1 -> OpComm2/3
  F2_MS_IN/1 -> OpComm2/2
  OpComm2/3 -> [F1_MS_IN]
  OpComm2/2 -> [F2_MS_IN]
  OpComm2/5 -> [F1_RELAY_OUT]
  OpComm2/4 -> [F2_RELAY_OUT]
  F1_RELAY_OUT/1 -> OpComm2/5
  F2_RELAY_OUT/1 -> OpComm2/4
  Memory1/1 -> LOAD_OUT/1
  Memory/1 -> F3_RELAY _OUT/1, [F3_RELAY_OUT]
  Bus Selector1/8 -> Generic_Relay_v2_8/1  "<F3_CB_8>"
  Bus Selector1/9 -> Generic_Relay_v2_9/1  "<F3_CB_9>"
  Generic_Relay_v2_9/1 -> Bus Creator6/9  "F3_CB_9"
  Generic_Relay_v2_8/1 -> Bus Creator6/8  "F3_CB_8"
  Modbus device8/1 -> Generic_Relay_v2_9/2
  Generic_Relay_v2_9/2 -> Modbus device8/1
  Generic_Relay_v2_8/2 -> Modbus device7/1
  Modbus device7/1 -> Generic_Relay_v2_8/2
  Bus Creator6/1 -> Memory/1
  Generic_Relay_v2_7/1 -> Bus Creator6/7  "F3_CB_7"
  Generic_Relay_v2_6/1 -> Bus Creator6/6  "F3_CB_6"
  Generic_Relay_v2_5/1 -> Bus Creator6/5  "F3_CB_5"
  Generic_Relay_v2_4/1 -> Bus Creator6/4  "F3_CB_4"
  Generic_Relay_v2_3/1 -> Bus Creator6/3  "F3_CB_3"
  Generic_Relay_v2_2/1 -> Bus Creator6/2  "F3_CB_2"
  Generic_Relay_v2_1/1 -> Bus Creator6/1  "F3_CB_1"
  Bus Selector1/7 -> Generic_Relay_v2_7/1  "<F3_CB_7>"
  Bus Selector1/6 -> Generic_Relay_v2_6/1  "<F3_CB_6>"
  Bus Selector1/5 -> Generic_Relay_v2_5/1  "<F3_CB_5>"
  Bus Selector1/4 -> Generic_Relay_v2_4/1  "<F3_CB_4>"
  Bus Selector1/3 -> Generic_Relay_v2_3/1  "<F3_CB_3>"
  Bus Selector1/2 -> Generic_Relay_v2_2/1  "<F3_CB_2>"
  Bus Selector1/1 -> Generic_Relay_v2_1/1  "<F3_CB_1>"
  F3_MS_IN/1 -> OpComm2/1
  Modbus device6/1 -> Generic_Relay_v2_7/2
  Generic_Relay_v2_7/2 -> Modbus device6/1
  Generic_Relay_v2_6/2 -> Modbus device5/1
  Modbus device5/1 -> Generic_Relay_v2_6/2
  Modbus device4/1 -> Generic_Relay_v2_5/2
  Generic_Relay_v2_5/2 -> Modbus device4/1
  Modbus device3/1 -> Generic_Relay_v2_4/2
  Generic_Relay_v2_4/2 -> Modbus device3/1
  Generic_Relay_v2_3/2 -> Modbus device2/1
  Modbus device2/1 -> Generic_Relay_v2_3/2
  Modbus device1/1 -> Generic_Relay_v2_2/2
  Generic_Relay_v2_2/2 -> Modbus device1/1
  Modbus device/1 -> Generic_Relay_v2_1/2
  Generic_Relay_v2_1/2 -> Modbus device/1
  OpComm2/1 -> [F3_MS_IN], Bus Selector1/1
  Load_Profiles/1 -> Memory1/1
